simulink model "signal_match"  (R2020b)
settings: Solver=VariableStepAuto  StartTime=0.0  StopTime=10.0  FixedStep=0.01  RelTol=1e-3
libraries: rllib x1, simulink x1
settings Model: SimulationMode=accelerator  Creator=callu  LastModifiedBy=callu

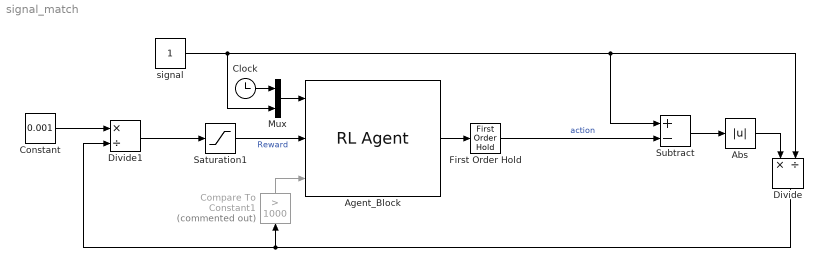
== system signal_match ==
  Abs : Abs
  Agent_Block : rllib/RL Agent  Agent=agent  ProvideReward=on  ProvideIsDone=on  ProvideCumRwd=off  TreatAsDirectFeedthrough=on  CollectLoggedSignals=on  CollectModelStates=on
  Clock : Clock
  Compare To Constant1 : simulink/Logic and Bit Operations/Compare To Constant  Commented=on  relop=>  const=1000  OutDataTypeStr=boolean
  Constant : Constant  Value=0.001
  Divide : Product  Inputs=*/
  Divide1 : Product  Inputs=*/
  First Order Hold : FirstOrderHold  ErrorTolerance=inf
  Mux : Mux  Inputs=2
  Saturation1 : Saturate  UpperLimit=1  LowerLimit=0
  Subtract : Sum  Inputs=+-
  signal : Constant
  wires:
  Compare To Constant1/1 -> Agent_Block/3
  Agent_Block/1 -> First Order Hold/1
  signal/1 -> Divide/2, Subtract/1, Mux/2
  Mux/1 -> Agent_Block/1
  Clock/1 -> Mux/1
  First Order Hold/1 -> Subtract/2  "action"
  Subtract/1 -> Abs/1
  Abs/1 -> Divide/1
  Divide/1 -> Compare To Constant1/1, Divide1/2
  Divide1/1 -> Saturation1/1
  Constant/1 -> Divide1/1
  Saturation1/1 -> Agent_Block/2  "Reward"
